simulink model "back_stoch"  (Simulink 8.9)
settings: Solver=ode3  StartTime=0.0  StopTime=10  RelTol=1e-3  EnableMultiTasking=on
undefined symbols (not defined in the file): sample_time
settings Model: Creator=paulghanem  LastModifiedBy=User
settings DataIOCC: SignalLoggingSaveFormat=Dataset
settings DebuggingCC: UnderspecifiedInitializationDetection=Simplified  MergeDetectMultiDrivingBlocksExec=error  SolverPrmCheckMsg=warning  FcnCallInpInsideContextMsg=error  StateNameClashWarn=none
settings GRTTargetCC: CombineOutputUpdateFcns=on  GRTInterface=off
settings ConfigComp: CovSFcnEnable=off

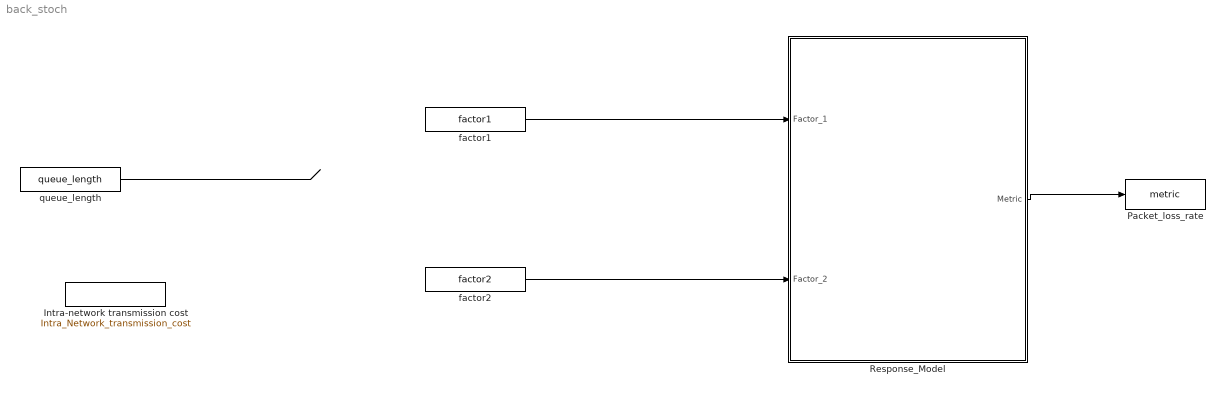
== system back_stoch ==
  "Intra-network transmission cost " : FromWorkspace  VariableName=Intra_Network_transmission_cost  SampleTime=sample_time
  "Packet_loss_rate " : ToWorkspace  VariableName=metric  SaveFormat=Structure With Time  SampleTime=-1
  Response_Model : MATLAB Function  TreatAsAtomicUnit=on
  factor1 : FromWorkspace  VariableName=factor1  SampleTime=sample_time
  "factor2 " : FromWorkspace  VariableName=factor2  SampleTime=sample_time
  queue_length : FromWorkspace  VariableName=queue_length  SampleTime=sample_time
  wires:
  Response_Model/1(Metric) -> "Packet_loss_rate "/1
  queue_length/1 -> ?
  factor1/1 -> Response_Model/1(Factor_1)
  "factor2 "/1 -> Response_Model/2(Factor_2)

== matlab function Response_Model ==
  data: Factor_1 input double; Metric output double; Factor_2 input double
function Metric = fcn(Factor_1, Factor_2)
%#codegen
Ts=1/500;
sig = 2e-4;
R = 1e-12*eye(7);
Rp = 1e-3*eye(7);
q1 = 1*eye(7);
q2 = 1e-2*eye(7);
Q = 0*[q1 zeros(7);zeros(7) q2];
H = [eye(7) Ts*eye(7);zeros(7) eye(7)];
I1 = [zeros(7);eye(7)];
I2 = [eye(7);zeros(7)];
F1 =  diag([0.20519,0.094428,0.094428,0.03,0.001,0.001,0.0003]);

   
 
 x11 = x1 + sig*(0.5 - rand(7,1));
 if t < 1
 e1=posd-x1;
 end
 e2=e1;
 
 posd=posd-e1;
 fposd=fposd-e1;
 
 
 
 
E = posd - x11;
Ed = fposd - x11;

K = Ts*I1'*P*inv(Ts^2*P + I1*Rp*I1' + (Ts*I2-I1)*R*(Ts*I2-I1)');
    K1 = 1*K(:,1:7);
    K2 = K(:,8:14);

 xx2=veld;
    Q22 = diag(diag(bq(xx2)*bq(xx2)'));
    Q = [zeros(7) zeros(7);zeros(7) Q22];
    PHI = H - Ts*I1*K;
    P1 = PHI*P*PHI' + I1*K*I1*Rp*I1'*K'*I1' + I1*K*(Ts*I2-I1)*R*(Ts*I2-I1)'*K'*I1' + Ts^2*I1*R*I1' + Ts^2*Q;
   
    
    
    ff = G(x11);   
    
     u= ff + (D(x11)+F1)*(faccd + K1*E + K2*(Ed - E)/Ts);
    
    %not to be used in real time
    U=u;
    
    x_1 =  x2*Ts + x1;
    x_2 = (-inv(D(x1)+F1)*(G(x1) + bq(x2)) + inv(D(x1)+F1)*U)*Ts + x2;
     
    
end 
function G=G(q)


DH_a = [0 0 0.045 -0.045 0 0 0];
    DH_d = [0 0 .55 0 0.45 0 0.061];
    DH_alpha = [-pi/2 pi/2 -pi/2 pi/2 -pi/2 pi/2 0];

    m = [10.7676 3.87 1.8022 2.4 0.1237 0.4979886 0.07548270];
    
     
    com= zeros(3,7);
    
   com(:,1) = [-0.00443422;0.12189039;-0.00066489];
    com(:,2) = [-0.00236983;0.03105614;0.01542114 ];
    com(:,3) = [-0.03825858;0.20750770;0.00003309];
    com(:,4) = [0.00498512;-0.00022942;0.13271662 ];
    com(:,5) = [0.00008921;0.00511217;0.00435824];
    com(:,6) = [-0.00012262;-0.01703194;0.02468336];
    com(:,7) = [-0.00007974;0.00016313;-0.00323552 ];
     
     % hand_mass =1.385;
      %  DH_d(7) =DH_d(7)+ .0953; % Adding the distance to the hand frame for the Schunk Gripper
       % com(:,7) =(com(:,7).*hand_mass+com(:,7).*m(7))/(hand_mass+m(7)); % Finding the combined center of mass
        %m(7) =m(7)+hand_mass;  
        
    I=zeros(3,3,7);
    T=zeros(4,4,7);
     I(:,:,1) = [0.29486350,-0.00795023,-0.00009311;
                 -0.00795023,0.11350017,-0.00018711;
                -0.00009311,-0.00018711,0.25065343];
    I(:,:,2) =[0.02606840,-0.00001346,-0.00011701;
               -0.00001346,0.01472202,0.00003659;
              -0.00011701,0.00003659,0.01934814];
    I(:,:,3) = [0.13671601,-0.01680434, 0.00000510;
               -0.01680434,0.00588354,-0.00000530;
                0.00000510,-0.00000530,0.13951371];
    I(:,:,4) = [ 0.05719268,0.00001467,0.00008193;
                 0.00001467,0.05716470,-0.00009417;
                 0.00008193,-0.00009417,0.00300441] ;
    I(:,:,5) =[0.00005587,0.00000026,.00000000;
               0.00000026,0.00007817,-0.00000083;
               0.00000000,-0.00000083,0.00006594];
    I(:,:,6) = [0.00093106,0.00000148,-0.00000201;
                0.00000148, 0.00049833,-0.00022162;
               -0.00000201,-0.00022162,0.00057483];
    I(:,:,7) = [0.003167342, 0,0;       % Approximate Inertia Tensor for Schunk Gripper
                0,0.001128942,0;
                 0,0,0.00258007;];  
            
             
for j=1:7,
        a = DH_a(j);
        d = DH_d(j);
        alpha = DH_alpha(j);
        T(:,:,j) = getTransformDH(a, d, alpha, q(j));
end 


comstar=zeros(4,7);

   
    comstar(:,1) = [com(:,1);1];
    comstar(:,2) = [com(:,2);1];
    comstar(:,3) = [com(:,3);1];
    comstar(:,4) = [com(:,4);1];
    comstar(:,5) = [com(:,5);1];
    comstar(:,6) = [com(:,6);1];
    comstar(:,7) = [com(:,7);1];
    
    Q=zeros(4,4);
    
    Q=[0,-1,0,0;
     1,0,0,0;
     0,0,0,0;
     0,0,0,0];
   
 gravity=[0,0,-9.81,0];
 G=zeros(7,1);
   G(1)= -m(1)*gravity*Q*T(:,:,1)*comstar(:,1)-m(2)*gravity*Q*T(:,:,1)*T(:,:,2)*comstar(:,2)-m(3)*gravity*Q*T(:,:,1)*T(:,:,2)*T(:,:,3)*comstar(:,3)-m(4)*gravity*Q*T(:,:,1)*T(:,:,2)*T(:,:,3)*T(:,:,4)*comstar(:,4)-m(5)*gravity*Q*T(:,:,1)*T(:,:,2)*T(:,:,3)*T(:,:,4)*T(:,:,5)*comstar(:,5)-m(6)*gravity*Q*T(:,:,1)*T(:,:,2)*T(:,:,3)*T(:,:,4)*T(:,:,5)*T(:,:,6)*comstar(:,6)-m(7)*gravity*Q*T(:,:,1)*T(:,:,2)*T(:,:,3)*T(:,:,4)*T(:,:,5)*T(:,:,6)*T(:,:,7)*comstar(:,7);   
   G(2)= -m(2)*gravity*T(:,:,1)*Q*T(:,:,2)*comstar(:,2)-m(3)*gravity*T(:,:,1)*Q*T(:,:,2)*T(:,:,3)*comstar(:,3)-m(4)*gravity*T(:,:,1)*Q*T(:,:,2)*T(:,:,3)*T(:,:,4)*comstar(:,4)-m(5)*gravity*T(:,:,1)*Q*T(:,:,2)*T(:,:,3)*T(:,:,4)*T(:,:,5)*comstar(:,5)-m(6)*gravity*T(:,:,1)*Q*T(:,:,2)*T(:,:,3)*T(:,:,4)*T(:,:,5)*T(:,:,6)*comstar(:,6)-m(7)*gravity*T(:,:,1)*Q*T(:,:,2)*T(:,:,3)*T(:,:,4)*T(:,:,5)*T(:,:,6)*T(:,:,7)*comstar(:,7);
   G(3)= -m(3)*gravity*T(:,:,1)*T(:,:,2)*Q*T(:,:,3)*comstar(:,3)-m(4)*gravity*T(:,:,1)*T(:,:,2)*Q*T(:,:,3)*T(:,:,4)*comstar(:,4)-m(5)*gravity*T(:,:,1)*T(:,:,2)*Q*T(:,:,3)*T(:,:,4)*T(:,:,5)*comstar(:,5)-m(6)*gravity*T(:,:,1)*T(:,:,2)*Q*T(:,:,3)*T(:,:,4)*T(:,:,5)*T(:,:,6)*comstar(:,6)-m(7)*gravity*T(:,:,1)*T(:,:,2)*Q*T(:,:,3)*T(:,:,4)*T(:,:,5)*T(:,:,6)*T(:,:,7)*comstar(:,7);
   G(4)= -m(4)*gravity*T(:,:,1)*T(:,:,2)*T(:,:,3)*Q*T(:,:,4)*comstar(:,4)-m(5)*gravity*T(:,:,1)*T(:,:,2)*T(:,:,3)*Q*T(:,:,4)*T(:,:,5)*comstar(:,5)-m(6)*gravity*T(:,:,1)*T(:,:,2)*T(:,:,3)*Q*T(:,:,4)*T(:,:,5)*T(:,:,6)*comstar(:,6)-m(7)*gravity*T(:,:,1)*T(:,:,2)*T(:,:,3)*Q*T(:,:,4)*T(:,:,5)*T(:,:,6)*T(:,:,7)*comstar(:,7);
   G(5)= -m(5)*gravity*T(:,:,1)*T(:,:,2)*T(:,:,3)*T(:,:,4)*Q*T(:,:,5)*comstar(:,5)-m(6)*gravity*T(:,:,1)*T(:,:,2)*T(:,:,3)*T(:,:,4)*Q*T(:,:,5)*T(:,:,6)*comstar(:,6)-m(7)*gravity*T(:,:,1)*T(:,:,2)*T(:,:,3)*T(:,:,4)*Q*T(:,:,5)*T(:,:,6)*T(:,:,7)*comstar(:,7);
   G(6)= -m(6)*gravity*T(:,:,1)*T(:,:,2)*T(:,:,3)*T(:,:,4)*T(:,:,5)*Q*T(:,:,6)*comstar(:,6)-m(7)*gravity*T(:,:,1)*T(:,:,2)*T(:,:,3)*T(:,:,4)*T(:,:,5)*Q*T(:,:,6)*T(:,:,7)*comstar(:,7);
   G(7)= -m(7)*gravity*T(:,:,1)*T(:,:,2)*T(:,:,3)*T(:,:,4)*T(:,:,5)*T(:,:,6)*Q*T(:,:,7)*comstar(:,7);
    
end 
    function T = getTransformDH(a,d,alpha,q)
    ct = cos(q);
    st = sin(q);
    cb = cos(alpha);
    sb = sin(alpha);
    
    T = [ ct, -st*cb,  st*sb, a*ct;
          st,  ct*cb, -ct*sb, a*st;
          0, sb, cb, d;
          0, 0, 0, 1 ];            
 end       
function bq = bq(qd)
 
 
 
s=20;
bc = [2.516; 2.581; 2.038; 0.956; 0.323; 0.315; 0.066];
B =  [1.142; 0.946; 0.309; 0.255; 0.025; 0.039; 0.004];
 
bq = bc.*atan(s*qd)*2/pi+B.*qd;
end 

function D =D(q);
DH_a = [0 0 0.045 -0.045 0 0 0];
    DH_d = [0 0 .55 0 0.45 0 0.061];
    DH_alpha = [-pi/2 pi/2 -pi/2 pi/2 -pi/2 pi/2 0];

    m = [10.7676 3.87 1.8022 2.4 0.1237 0.4979886 0.07548270];
    
     
    com= zeros(3,7);
    
   com(:,1) = [-0.00443422;0.12189039;-0.00066489];
    com(:,2) = [-0.00236983;0.03105614;0.01542114 ];
    com(:,3) = [-0.03825858;0.20750770;0.00003309];
    com(:,4) = [0.00498512;-0.00022942;0.13271662 ];
    com(:,5) = [0.00008921;0.00511217;0.00435824];
    com(:,6) = [-0.00012262;-0.01703194;0.02468336];
    com(:,7) = [-0.00007974;0.00016313;-0.00323552 ];
     
       
        
    I=zeros(3,3,7);
    T=zeros(4,4,7);
     I(:,:,1) = [0.29486350,-0.00795023,-0.00009311;
                 -0.00795023,0.11350017,-0.00018711;
                -0.00009311,-0.00018711,0.25065343];
    I(:,:,2) =[0.02606840,-0.00001346,-0.00011701;
               -0.00001346,0.01472202,0.00003659;
              -0.00011701,0.00003659,0.01934814];
    I(:,:,3) = [0.13671601,-0.01680434, 0.00000510;
               -0.01680434,0.00588354,-0.00000530;
                0.00000510,-0.00000530,0.13951371];
    I(:,:,4) = [ 0.05719268,0.00001467,0.00008193;
                 0.00001467,0.05716470,-0.00009417;
                 0.00008193,-0.00009417,0.00300441] ;
    I(:,:,5) =[0.00005587,0.00000026,.00000000;
               0.00000026,0.00007817,-0.00000083;
               0.00000000,-0.00000083,0.00006594];
    I(:,:,6) = [0.00093106,0.00000148,-0.00000201;
                0.00000148, 0.00049833,-0.00022162;
               -0.00000201,-0.00022162,0.00057483];
    I(:,:,7) = [0.003167342, 0,0;       % Approximate Inertia Tensor for Schunk Gripper
                0,0.001128942,0;
                 0,0,0.00258007;];  
            
             
             
for j=1:7,
        a = DH_a(j);
        d = DH_d(j);
        alpha = DH_alpha(j);
        T(:,:,j) = getTransformDH(a, d, alpha, q(j));
end 

comstar=zeros(4,7);

   
    comstar(:,1) = [com(:,1);1];
    comstar(:,2) = [com(:,2);1];
    comstar(:,3) = [com(:,3);1];
    comstar(:,4) = [com(:,4);1];
    comstar(:,5) = [com(:,5);1];
    comstar(:,6) = [com(:,6);1];
    comstar(:,7) = [com(:,7);1];
    
    Q=zeros(4,4);
    
    Q=[0,-1,0,0;
     1,0,0,0;
     0,0,0,0;
     0,0,0,0];
   

   
U=zeros(4,4,7,7);
   
   U(:,:,1,1)= Q*T(:,:,1);
   U(:,:,2,1)= Q*T(:,:,1)*T(:,:,2);
   U(:,:,3,1)= Q*T(:,:,1)*T(:,:,2)*T(:,:,3);
   U(:,:,4,1)= Q*T(:,:,1)*T(:,:,2)*T(:,:,3)*T(:,:,4);
   U(:,:,5,1)= Q*T(:,:,1)*T(:,:,2)*T(:,:,3)*T(:,:,4)*T(:,:,5);
   U(:,:,6,1)= Q*T(:,:,1)*T(:,:,2)*T(:,:,3)*T(:,:,4)*T(:,:,5)*T(:,:,6);
   U(:,:,7,1)= Q*T(:,:,1)*T(:,:,2)*T(:,:,3)*T(:,:,4)*T(:,:,5)*T(:,:,6)*T(:,:,7);
   
   
   U(:,:,2,2)= T(:,:,1)*Q*T(:,:,2);
   U(:,:,3,2)= T(:,:,1)*Q*T(:,:,2)*T(:,:,3);
   U(:,:,4,2)= T(:,:,1)*Q*T(:,:,2)*T(:,:,3)*T(:,:,4);
   U(:,:,5,2)= T(:,:,1)*Q*T(:,:,2)*T(:,:,3)*T(:,:,4)*T(:,:,5);
   U(:,:,6,2)= T(:,:,1)*Q*T(:,:,2)*T(:,:,3)*T(:,:,4)*T(:,:,5)*T(:,:,6);
   U(:,:,7,2)= T(:,:,1)*Q*T(:,:,2)*T(:,:,3)*T(:,:,4)*T(:,:,5)*T(:,:,6)*T(:,:,7);
   
  
   U(:,:,3,3)= T(:,:,1)*T(:,:,2)*Q*T(:,:,3);
   U(:,:,4,3)= T(:,:,1)*T(:,:,2)*Q*T(:,:,3)*T(:,:,4);
   U(:,:,5,3)= T(:,:,1)*T(:,:,2)*Q*T(:,:,3)*T(:,:,4)*T(:,:,5);
   U(:,:,6,3)= T(:,:,1)*T(:,:,2)*Q*T(:,:,3)*T(:,:,4)*T(:,:,5)*T(:,:,6);
   U(:,:,7,3)= T(:,:,1)*T(:,:,2)*Q*T(:,:,3)*T(:,:,4)*T(:,:,5)*T(:,:,6)*T(:,:,7);
   
   U(:,:,4,4)= T(:,:,1)*T(:,:,2)*T(:,:,3)*Q*T(:,:,4);
   U(:,:,5,4)= T(:,:,1)*T(:,:,2)*T(:,:,3)*Q*T(:,:,4)*T(:,:,5);
   U(:,:,6,4)= T(:,:,1)*T(:,:,2)*T(:,:,3)*Q*T(:,:,4)*T(:,:,5)*T(:,:,6);
   U(:,:,7,4)= T(:,:,1)*T(:,:,2)*T(:,:,3)*Q*T(:,:,4)*T(:,:,5)*T(:,:,6)*T(:,:,7);
   
   U(:,:,5,5)= T(:,:,1)*T(:,:,2)*T(:,:,3)*T(:,:,4)*Q*T(:,:,5);
   U(:,:,6,5)= T(:,:,1)*T(:,:,2)*T(:,:,3)*T(:,:,4)*Q*T(:,:,5)*T(:,:,6);
   U(:,:,7,5)= T(:,:,1)*T(:,:,2)*T(:,:,3)*T(:,:,4)*Q*T(:,:,5)*T(:,:,6)*T(:,:,7);
   
   U(:,:,6,6)= T(:,:,1)*T(:,:,2)*T(:,:,3)*T(:,:,4)*T(:,:,5)*Q*T(:,:,6);
   U(:,:,7,6)= T(:,:,1)*T(:,:,2)*T(:,:,3)*T(:,:,4)*T(:,:,5)*Q*T(:,:,6)*T(:,:,7);
   
   U(:,:,7,7)= T(:,:,1)*T(:,:,2)*T(:,:,3)*T(:,:,4)*T(:,:,5)*T(:,:,6)*Q*T(:,:,7);
   
   
   
  
   J=zeros(4,4,7);
 
   
   J(:,:,1)=[0.5*(-I(1,1,1)+I(2,2,1)+I(3,3,1)), I(1,2,1), I(1,3,1), m(1)*com(1,1);
             I(1,2,1) ,0.5*(I(1,1,1)-I(2,2,1)+I(3,3,1)), I(2,3,1), m(1)*com(2,1);
             I(1,3,1), I(2,3,1), 0.5*(I(1,1,1)+I(2,2,1)-I(3,3,1)), m(1)*com(3,1);
              m(1)*com(1,1), m(1)*com(2,1), m(1)*com(3,1), m(1)];
   
    J(:,:,2)=[0.5*(-I(1,1,2)+I(2,2,2)+I(3,3,2)), I(1,2,2), I(1,3,2), m(2)*com(1,2);
             I(1,2,2) ,0.5*(I(1,1,2)-I(2,2,2)+I(3,3,2)), I(2,3,2), m(2)*com(2,2);
             I(1,3,2), I(2,3,2), 0.5*(I(1,1,2)+I(2,2,2)-I(3,3,2)), m(2)*com(3,2);
              m(2)*com(1,2), m(2)*com(2,2), m(2)*com(3,2), m(2)];
   
          
     J(:,:,3)=[0.5*(-I(1,1,3)+I(2,2,3)+I(3,3,3)), I(1,2,3), I(1,3,3), m(3)*com(1,3);
             I(1,2,3) ,0.5*(I(1,1,3)-I(2,2,3)+I(3,3,3)), I(2,3,3), m(3)*com(2,3);
             I(1,3,3), I(2,3,3), 0.5*(I(1,1,3)+I(2,2,3)-I(3,3,3)), m(3)*com(3,3);
              m(3)*com(1,3), m(3)*com(2,3), m(3)*com(3,3), m(3)];      
   
   
    J(:,:,4)=[0.5*(-I(1,1,4)+I(2,2,4)+I(3,3,4)), I(1,2,4), I(1,3,4), m(4)*com(1,4);
             I(1,2,4) ,0.5*(I(1,1,4)-I(2,2,4)+I(3,3,4)), I(2,3,4), m(4)*com(2,4);
             I(1,3,4), I(2,3,4), 0.5*(I(1,1,4)+I(2,2,4)-I(3,3,4)), m(4)*com(3,4);
              m(4)*com(1,4), m(4)*com(2,4), m(4)*com(3,4), m(4)];
   
   
    J(:,:,5)=[0.5*(-I(1,1,5)+I(2,2,5)+I(3,3,5)), I(1,2,5), I(1,3,5), m(5)*com(1,5);
             I(1,2,5) ,0.5*(I(1,1,5)-I(2,2,5)+I(3,3,5)), I(2,3,5), m(5)*com(2,5);
             I(1,3,5), I(2,3,5), 0.5*(I(1,1,5)+I(2,2,5)-I(3,3,5)), m(5)*com(3,5);
              m(5)*com(1,5), m(5)*com(2,5), m(5)*com(3,5), m(5)];
   
   
    J(:,:,6)=[0.5*(-I(1,1,6)+I(2,2,6)+I(3,3,6)), I(1,2,6), I(1,3,6), m(6)*com(1,6);
             I(1,2,6) ,0.5*(I(1,1,6)-I(2,2,6)+I(3,3,6)), I(2,3,6), m(6)*com(2,6);
             I(1,3,6), I(2,3,6), 0.5*(I(1,1,6)+I(2,2,6)-I(3,3,6)), m(6)*com(3,6);
              m(6)*com(1,6), m(6)*com(2,6), m(6)*com(3,6), m(6)];
   
   
    J(:,:,7)=[0.5*(-I(1,1,7)+I(2,2,7)+I(3,3,7)), I(1,2,7), I(1,3,7), m(7)*com(1,7);
             I(1,2,7) ,0.5*(I(1,1,7)-I(2,2,7)+I(3,3,7)), I(2,3,7), m(7)*com(2,7);
             I(1,3,7), I(2,3,7), 0.5*(I(1,1,7)+I(2,2,7)-I(3,3,7)), m(7)*com(3,7);
              m(7)*com(1,7), m(7)*com(2,7), m(7)*com(3,7), m(7)];
          
          D=zeros(7,7);
   
   
    D(1,1)= trace(U(:,:,1,1)*J(:,:,1)*transpose(U(:,:,1,1))) + trace(U(:,:,2,1)*J(:,:,2)*transpose(U(:,:,2,1))) + trace(U(:,:,3,1)*J(:,:,3)*transpose(U(:,:,3,1))) + trace(U(:,:,4,1)*J(:,:,4)*transpose(U(:,:,4,1))) + trace(U(:,:,5,1)*J(:,:,5)*transpose(U(:,:,5,1))) + trace(U(:,:,6,1)*J(:,:,6)*transpose(U(:,:,6,1))) + trace(U(:,:,7,1)*J(:,:,7)*transpose(U(:,:,7,1))) ;
    D(1,2)= trace(U(:,:,2,2)*J(:,:,2)*transpose(U(:,:,2,1))) + trace(U(:,:,3,2)*J(:,:,3)*transpose(U(:,:,3,1))) + trace(U(:,:,4,2)*J(:,:,4)*transpose(U(:,:,4,1))) +trace(U(:,:,5,2)*J(:,:,5)*transpose(U(:,:,5,1))) + trace(U(:,:,6,2)*J(:,:,6)*transpose(U(:,:,6,1))) + trace(U(:,:,7,2)*J(:,:,7)*transpose(U(:,:,7,1))); 
    D(1,3)= trace(U(:,:,3,3)*J(:,:,3)*transpose(U(:,:,3,1)))+ trace(U(:,:,4,3)*J(:,:,4)*transpose(U(:,:,4,1)))+ trace(U(:,:,5,3)*J(:,:,5)*transpose(U(:,:,5,1)))+ trace(U(:,:,6,3)*J(:,:,6)*transpose(U(:,:,6,1)))+ trace(U(:,:,7,3)*J(:,:,7)*transpose(U(:,:,7,1))); 
    D(1,4)= trace(U(:,:,4,4)*J(:,:,4)*transpose(U(:,:,4,1)))+ trace(U(:,:,5,4)*J(:,:,5)*transpose(U(:,:,5,1)))+ trace(U(:,:,6,4)*J(:,:,6)*transpose(U(:,:,6,1)))+ trace(U(:,:,7,4)*J(:,:,7)*transpose(U(:,:,7,1)));
    D(1,5)= trace(U(:,:,5,5)*J(:,:,5)*transpose(U(:,:,5,1)))+ trace(U(:,:,6,5)*J(:,:,6)*transpose(U(:,:,6,1)))+ trace(U(:,:,7,5)*J(:,:,7)*transpose(U(:,:,7,1)));
    D(1,6)= trace(U(:,:,6,6)*J(:,:,6)*transpose(U(:,:,6,1)))+ trace(U(:,:,7,6)*J(:,:,7)*transpose(U(:,:,7,1)));
    D(1,7)= trace(U(:,:,7,7)*J(:,:,7)*transpose(U(:,:,7,1)));
    
    D(2,1)= trace(U(:,:,2,1)*J(:,:,2)*transpose(U(:,:,2,2)))+ trace(U(:,:,3,1)*J(:,:,3)*transpose(U(:,:,3,2)))+ trace(U(:,:,4,1)*J(:,:,4)*transpose(U(:,:,4,2)))+ trace(U(:,:,5,1)*J(:,:,5)*transpose(U(:,:,5,2)))+ trace(U(:,:,6,1)*J(:,:,6)*transpose(U(:,:,6,2)))+ trace(U(:,:,7,1)*J(:,:,7)*transpose(U(:,:,7,2)));
    D(2,2)= trace(U(:,:,2,2)*J(:,:,2)*transpose(U(:,:,2,2)))+ trace(U(:,:,3,2)*J(:,:,3)*transpose(U(:,:,3,2)))+ trace(U(:,:,4,2)*J(:,:,4)*transpose(U(:,:,4,2)))+ trace(U(:,:,5,2)*J(:,:,5)*transpose(U(:,:,5,2)))+ trace(U(:,:,6,2)*J(:,:,6)*transpose(U(:,:,6,2)))+ trace(U(:,:,7,2)*J(:,:,7)*transpose(U(:,:,7,2)));
    D(2,3)= trace(U(:,:,3,3)*J(:,:,3)*transpose(U(:,:,3,2)))+ trace(U(:,:,4,3)*J(:,:,4)*transpose(U(:,:,4,2)))+ trace(U(:,:,5,3)*J(:,:,5)*transpose(U(:,:,5,2)))+ trace(U(:,:,6,3)*J(:,:,6)*transpose(U(:,:,6,2)))+ trace(U(:,:,7,3)*J(:,:,7)*transpose(U(:,:,7,2))); 
    D(2,4)= trace(U(:,:,4,4)*J(:,:,4)*transpose(U(:,:,4,2)))+ trace(U(:,:,5,4)*J(:,:,5)*transpose(U(:,:,5,2)))+ trace(U(:,:,6,4)*J(:,:,6)*transpose(U(:,:,6,2)))+ trace(U(:,:,7,4)*J(:,:,7)*transpose(U(:,:,7,2))); 
    D(2,5)= trace(U(:,:,5,5)*J(:,:,5)*transpose(U(:,:,5,2)))+ trace(U(:,:,6,5)*J(:,:,6)*transpose(U(:,:,6,2)))+ trace(U(:,:,7,5)*J(:,:,7)*transpose(U(:,:,7,2)));
    D(2,6)= trace(U(:,:,6,6)*J(:,:,6)*transpose(U(:,:,6,2)))+ trace(U(:,:,7,6)*J(:,:,7)*transpose(U(:,:,7,2))); 
    D(2,7)= trace(U(:,:,7,7)*J(:,:,7)*transpose(U(:,:,7,2)));
  
    D(3,1)= trace(U(:,:,3,1)*J(:,:,3)*transpose(U(:,:,3,3)))+ trace(U(:,:,4,1)*J(:,:,4)*transpose(U(:,:,4,3)))+ trace(U(:,:,5,1)*J(:,:,5)*transpose(U(:,:,5,3)))+ trace(U(:,:,6,1)*J(:,:,6)*transpose(U(:,:,6,3)))+ trace(U(:,:,7,1)*J(:,:,7)*transpose(U(:,:,7,3)));
    D(3,2)= trace(U(:,:,3,2)*J(:,:,3)*transpose(U(:,:,3,3)))+ trace(U(:,:,4,2)*J(:,:,4)*transpose(U(:,:,4,3)))+ trace(U(:,:,5,2)*J(:,:,5)*transpose(U(:,:,5,3)))+ trace(U(:,:,6,2)*J(:,:,6)*transpose(U(:,:,6,3)))+ trace(U(:,:,7,2)*J(:,:,7)*transpose(U(:,:,7,3)));
    D(3,3)= trace(U(:,:,3,3)*J(:,:,3)*transpose(U(:,:,3,3)))+ trace(U(:,:,4,3)*J(:,:,4)*transpose(U(:,:,4,3)))+ trace(U(:,:,5,3)*J(:,:,5)*transpose(U(:,:,5,3)))+ trace(U(:,:,6,3)*J(:,:,6)*transpose(U(:,:,6,3)))+ trace(U(:,:,7,3)*J(:,:,7)*transpose(U(:,:,7,3)));
    D(3,4)= trace(U(:,:,4,4)*J(:,:,4)*transpose(U(:,:,4,3)))+ trace(U(:,:,5,4)*J(:,:,5)*transpose(U(:,:,5,3)))+ trace(U(:,:,6,4)*J(:,:,6)*transpose(U(:,:,6,3)))+ trace(U(:,:,7,4)*J(:,:,7)*transpose(U(:,:,7,3)));
    D(3,5)= trace(U(:,:,5,5)*J(:,:,5)*transpose(U(:,:,5,3)))+ trace(U(:,:,6,5)*J(:,:,6)*transpose(U(:,:,6,3)))+ trace(U(:,:,7,5)*J(:,:,7)*transpose(U(:,:,7,3)));
    D(3,6)= trace(U(:,:,6,6)*J(:,:,6)*transpose(U(:,:,6,3)))+ trace(U(:,:,7,6)*J(:,:,7)*transpose(U(:,:,7,3)));
    D(3,7)= trace(U(:,:,7,7)*J(:,:,7)*transpose(U(:,:,7,3)));
     
     
    D(4,1)= trace(U(:,:,4,1)*J(:,:,4)*transpose(U(:,:,4,4)))+ trace(U(:,:,5,1)*J(:,:,5)*transpose(U(:,:,5,4)))+ trace(U(:,:,6,1)*J(:,:,6)*transpose(U(:,:,6,4)))+ trace(U(:,:,7,1)*J(:,:,7)*transpose(U(:,:,7,4))); 
    D(4,2)= trace(U(:,:,4,2)*J(:,:,4)*transpose(U(:,:,4,4)))+ trace(U(:,:,5,2)*J(:,:,5)*transpose(U(:,:,5,4)))+ trace(U(:,:,6,2)*J(:,:,6)*transpose(U(:,:,6,4)))+ trace(U(:,:,7,2)*J(:,:,7)*transpose(U(:,:,7,4))); 
    D(4,3)= trace(U(:,:,4,3)*J(:,:,4)*transpose(U(:,:,4,4)))+ trace(U(:,:,5,3)*J(:,:,5)*transpose(U(:,:,5,4)))+ trace(U(:,:,6,3)*J(:,:,6)*transpose(U(:,:,6,4)))+ trace(U(:,:,7,3)*J(:,:,7)*transpose(U(:,:,7,4)));
    D(4,4)= trace(U(:,:,4,4)*J(:,:,4)*transpose(U(:,:,4,4)))+ trace(U(:,:,5,4)*J(:,:,5)*transpose(U(:,:,5,4)))+ trace(U(:,:,6,4)*J(:,:,6)*transpose(U(:,:,6,4)))+ trace(U(:,:,7,4)*J(:,:,7)*transpose(U(:,:,7,4)));
    D(4,5)= trace(U(:,:,5,5)*J(:,:,5)*transpose(U(:,:,5,4)))+ trace(U(:,:,6,5)*J(:,:,6)*transpose(U(:,:,6,4)))+ trace(U(:,:,7,5)*J(:,:,7)*transpose(U(:,:,7,4)));
    D(4,6)= trace(U(:,:,6,6)*J(:,:,6)*transpose(U(:,:,6,4)))+ trace(U(:,:,7,6)*J(:,:,7)*transpose(U(:,:,7,4))); 
    D(4,7)= trace(U(:,:,7,7)*J(:,:,7)*transpose(U(:,:,7,4)));
    
    D(5,1)= trace(U(:,:,5,1)*J(:,:,5)*transpose(U(:,:,5,5)))+ trace(U(:,:,6,1)*J(:,:,6)*transpose(U(:,:,6,5)))+ trace(U(:,:,7,1)*J(:,:,7)*transpose(U(:,:,7,5)));
    D(5,2)= trace(U(:,:,5,2)*J(:,:,5)*transpose(U(:,:,5,5)))+ trace(U(:,:,6,2)*J(:,:,6)*transpose(U(:,:,6,5)))+ trace(U(:,:,7,2)*J(:,:,7)*transpose(U(:,:,7,5)));
    D(5,3)= trace(U(:,:,5,3)*J(:,:,5)*transpose(U(:,:,5,5)))+ trace(U(:,:,6,3)*J(:,:,6)*transpose(U(:,:,6,5)))+ trace(U(:,:,7,3)*J(:,:,7)*transpose(U(:,:,7,5))); 
    D(5,4)= trace(U(:,:,5,4)*J(:,:,5)*transpose(U(:,:,5,5)))+ trace(U(:,:,6,4)*J(:,:,6)*transpose(U(:,:,6,5)))+ trace(U(:,:,7,4)*J(:,:,7)*transpose(U(:,:,7,5))); 
    D(5,5)= trace(U(:,:,5,5)*J(:,:,5)*transpose(U(:,:,5,5)))+ trace(U(:,:,6,5)*J(:,:,6)*transpose(U(:,:,6,5)))+ trace(U(:,:,7,5)*J(:,:,7)*transpose(U(:,:,7,5)));
    D(5,6)= trace(U(:,:,6,6)*J(:,:,6)*transpose(U(:,:,6,5)))+ trace(U(:,:,7,6)*J(:,:,7)*transpose(U(:,:,7,5))); 
    D(5,7)= trace(U(:,:,7,7)*J(:,:,7)*transpose(U(:,:,7,5)));
    
    D(6,1)= trace(U(:,:,6,1)*J(:,:,6)*transpose(U(:,:,6,6)))+ trace(U(:,:,7,1)*J(:,:,7)*transpose(U(:,:,7,6)));
    D(6,2)= trace(U(:,:,6,2)*J(:,:,6)*transpose(U(:,:,6,6)))+ trace(U(:,:,7,2)*J(:,:,7)*transpose(U(:,:,7,6)));
    D(6,3)= trace(U(:,:,6,3)*J(:,:,6)*transpose(U(:,:,6,6)))+ trace(U(:,:,7,3)*J(:,:,7)*transpose(U(:,:,7,6))); 
    D(6,4)= trace(U(:,:,6,4)*J(:,:,6)*transpose(U(:,:,6,6)))+ trace(U(:,:,7,4)*J(:,:,7)*transpose(U(:,:,7,6))); 
    D(6,5)= trace(U(:,:,6,5)*J(:,:,6)*transpose(U(:,:,6,6)))+ trace(U(:,:,7,5)*J(:,:,7)*transpose(U(:,:,7,6))); 
    D(6,6)= trace(U(:,:,6,6)*J(:,:,6)*transpose(U(:,:,6,6)))+ trace(U(:,:,7,6)*J(:,:,7)*transpose(U(:,:,7,6))); 
    D(6,7)= trace(U(:,:,7,7)*J(:,:,7)*transpose(U(:,:,7,6)));
    
    D(7,1)= trace(U(:,:,7,1)*J(:,:,7)*transpose(U(:,:,7,7)));
    D(7,2)= trace(U(:,:,7,2)*J(:,:,7)*transpose(U(:,:,7,7)));
    D(7,3)= trace(U(:,:,7,3)*J(:,:,7)*transpose(U(:,:,7,7)));
    D(7,4)= trace(U(:,:,7,4)*J(:,:,7)*transpose(U(:,:,7,7)));
    D(7,5)= trace(U(:,:,7,5)*J(:,:,7)*transpose(U(:,:,7,7)));
    D(7,6)= trace(U(:,:,7,6)*J(:,:,7)*transpose(U(:,:,7,7)));
    D(7,7)= trace(U(:,:,7,7)*J(:,:,7)*transpose(U(:,:,7,7)));
end
